simulink model "PI_Laengsregler_2"  (R2019b)
settings: Solver=VariableStepAuto  StartTime=0.0  StopTime=50  FixedStep=1e-6  MaxStep=1e-4  RelTol=1e-3
values from neighbouring files (symbols this model uses):
  A = [a11, a12, a13, a14, a15; a21, a22, a23, a24, a25; a31, a32, a33, a34,     a35; a41, a42, a43, a44, a45; a51, a52, a53, a54, a55]    [initial_data.m]
  i = 1    [initial_data.m]
  v = 9    [initial_data.m]
undefined symbols (not defined in the file or in its folder): b, cT, p, tau, Ur
libraries: cstblocks x1

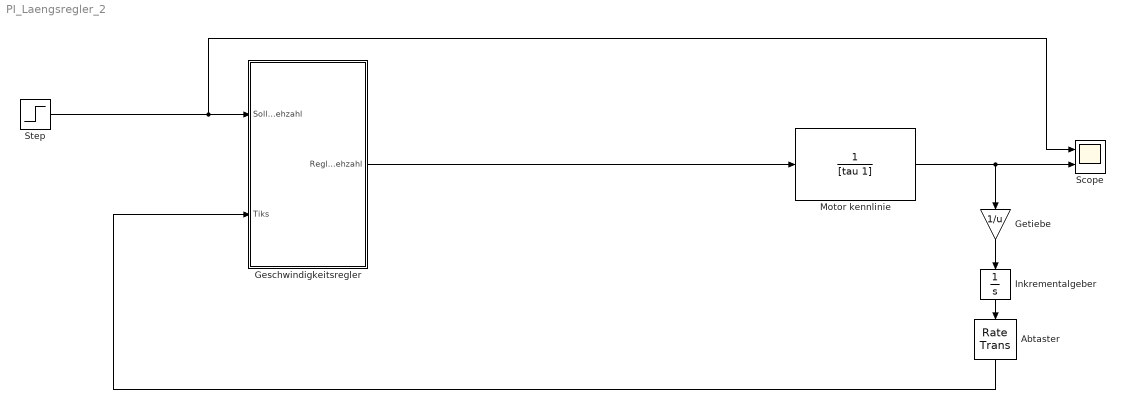
== system PI_Laengsregler_2 ==
  Abtaster : RateTransition  OutPortSampleTime=tasten
  "Geschwindigkeitsregler " : Subsystem
  Getiebe : Gain  Gain=1/u
  Inkrementalgeber : Integrator
  Motor kennlinie : TransferFcn  Denominator=[tau 1]
  Scope : Scope  NumInputPorts=2
  Step : Step  After=u*v/Ur  SampleTime=0
  wires:
  Inkrementalgeber/1 -> Abtaster/1
  Motor kennlinie/1 -> Getiebe/1, Scope/2
  Step/1 -> Scope/1, "Geschwindigkeitsregler "/1("Sollmotordrehzahl ")
  "Geschwindigkeitsregler "/1(Reglermotordrehzahl) -> Motor kennlinie/1
  Abtaster/1 -> "Geschwindigkeitsregler "/2(Tiks)
  Getiebe/1 -> Inkrementalgeber/1

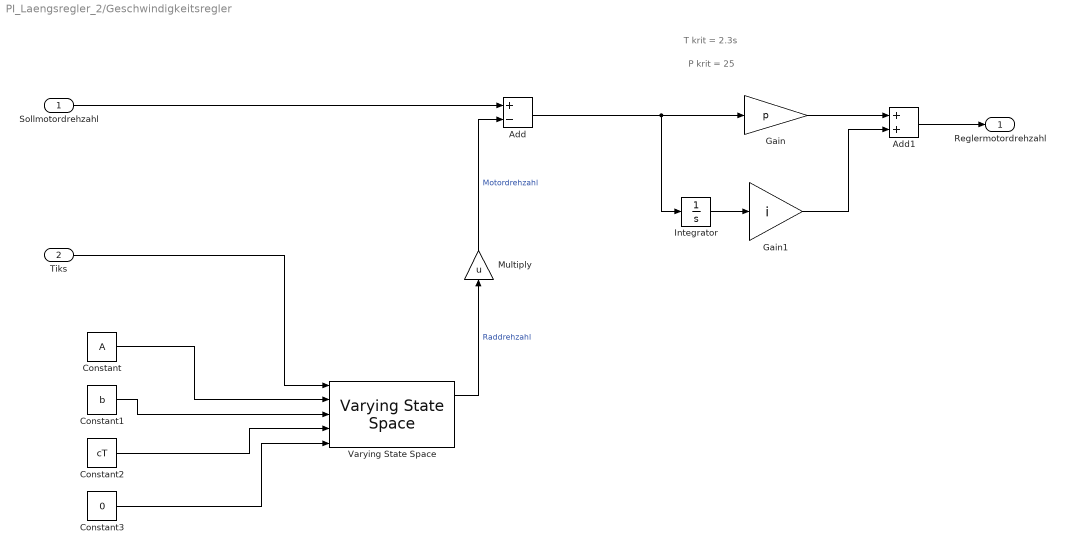
== system PI_Laengsregler_2/Geschwindigkeitsregler  ==
  note: T krit = 2.3s
  note: P krit = 25
  "Sollmotordrehzahl " : Inport
  Tiks : Inport  Port=2
  Add : Sum  Inputs=+-
  Add1 : Sum
  Constant : Constant  Value=A  VectorParams1D=off
  Constant1 : Constant  Value=b  VectorParams1D=off
  Constant2 : Constant  Value=cT  VectorParams1D=off
  Constant3 : Constant  Value=0
  Gain : Gain  Gain=p
  Gain1 : Gain  Gain=i
  Integrator : Integrator
  Multiply : Gain  Gain=u
  Varying State Space : cstblocks/Linear Parameter Varying/Varying State Space  x0=0  xNames=''  OutputX=on  OutputDX=on
  Reglermotordrehzahl : Outport
  wires:
  Add/1 -> Integrator/1, Gain/1
  Constant2/1 -> Varying State Space/4
  Integrator/1 -> Gain1/1
  Constant3/1 -> Varying State Space/5
  Constant1/1 -> Varying State Space/3
  Gain1/1 -> Add1/2
  Gain/1 -> Add1/1
  Varying State Space/1 -> Multiply/1  "Raddrehzahl"
  Constant/1 -> Varying State Space/2
  Add1/1 -> Reglermotordrehzahl/1
  "Sollmotordrehzahl "/1 -> Add/1
  Tiks/1 -> Varying State Space/1
  Multiply/1 -> Add/2  "Motordrehzahl"
